simulink model "example_F27_second_attempt"  (R2016b)
settings: Solver=VariableStepAuto  StartTime=0.0  StopTime=50.0  RelTol=1e-3
PreLoadFcn:
  | k = 20;
  | m = 90;
  | Cviscous = 1;
  | Cdrag = 1;
  | g = 9.81;
settings Model: Creator=training-ah  LastModifiedBy=training-ah

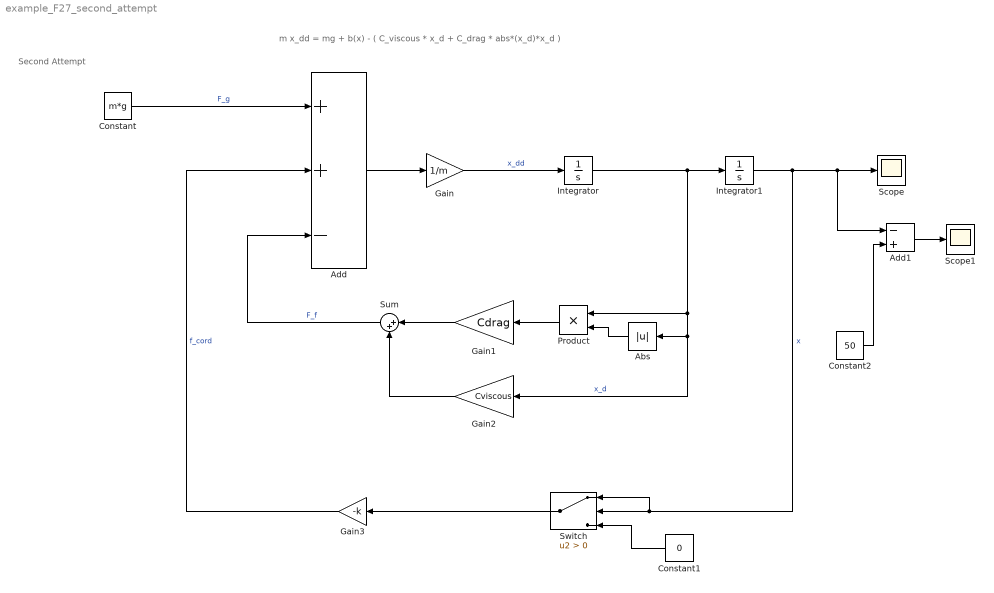
== system example_F27_second_attempt ==
  note: Second Attempt
  note: m x_dd = mg + b(x) - ( C_viscous * x_d + C_drag * abs*(x_d)*x_d )
  Abs : Abs
  Add : Sum  Inputs=++-
  Add1 : Sum  Inputs=-+
  Constant : Constant  Value=m*g
  Constant1 : Constant  Value=0
  Constant2 : Constant  Value=50
  Gain : Gain  Gain=1/m
  Gain1 : Gain  Gain=Cdrag
  Gain2 : Gain  Gain=Cviscous
  Gain3 : Gain  Gain=-k
  Integrator : Integrator
  Integrator1 : Integrator  InitialCondition=-30
  Product : Product
  Scope : Scope
  Scope1 : Scope
  Sum : Sum  Inputs=|++
  Switch : Switch  Criteria=u2 > Threshold
  wires:
  Gain/1 -> Integrator/1  "x_dd"
  Integrator/1 -> Integrator1/1, Gain2/1, Abs/1, Product/1  "x_d"
  Integrator1/1 -> Switch/1, Switch/2, Add1/1, Scope/1  "x"
  Constant/1 -> Add/1  "F_g"
  Add/1 -> Gain/1
  Abs/1 -> Product/2
  Product/1 -> Gain1/1
  Gain1/1 -> Sum/1
  Gain2/1 -> Sum/2
  Sum/1 -> Add/3  "F_f"
  Constant1/1 -> Switch/3
  Switch/1 -> Gain3/1
  Gain3/1 -> Add/2  "f_cord"
  Constant2/1 -> Add1/2
  Add1/1 -> Scope1/1
